simulink model "subsystem_118_bus_self_clearing_blocking"  (R2025b)
settings: Solver=ode45  StartTime=0.0  StopTime=Tstop  FixedStep=Ts  RelTol=1e-12  AbsTol=1e-12
values from neighbouring files (symbols this model uses):
  gfl3_enable_before = ones(numberOfGFLs,1)    [plotFun.m]
  gfl3_enable_blocked = gfl3_enable_before    [plotFun.m]
  gfl3_enable_clear_increment = gfl3_enable_before - gfl3_enable_blocked    [plotFun.m]
  gfl3_enable_zero = zeros(numberOfGFLs,1)    [plotFun.m]
  Imax = 15    [config_file.m]
  nominalInter =     [nominalInter.mat]
  nominalU =     [nominalU.mat]
  nominalY =     [nominalY.mat]
  P_input = 0    [main_sub_118_bus.m]    (also in plotFun.m = 0.03)
  sub = struct    [main_sub_118_bus.m]
  sys_j = sys_j(1:end-1)    [IBR_modelGenerator.m]
  sys_j_AA = sys_j    [modularMOR_main.m]
  sys_j_BT = sys_j    [modularMOR_main.m]
  Tclear_gfl = 0.11    [plotFun.m]
  Tstep_gfl = 0.1    [main_sub_118_bus.m]
  Tstep_gfm = 0.1    [main_sub_118_bus.m]
  Ttrip_gfl = 0.1    [plotFun.m]
  w = 2*pi*50    (= 314.159265359)    [config_file.m]    (also in mirrorMimoWeightedFrequencyData.m = w(:); modularMOR_main.m = w(:).'; plotTest.m = w(:).')
undefined symbols (not defined in the file or in its folder): con_sub, linSys1, linSys2, linSys3
libraries: simulink x10
(part 1 of 7)
settings Model: Creator=mj419  LastModifiedBy=hz1021
settings OptimizationCC: ReuseModelBlockBuffer=off
settings RTWCC: GPUComputeCapability=3.5

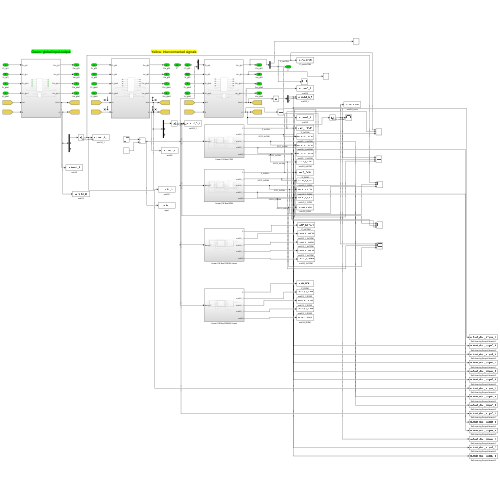
[thumbnail: Simulink's stored preview of the top-level diagram]
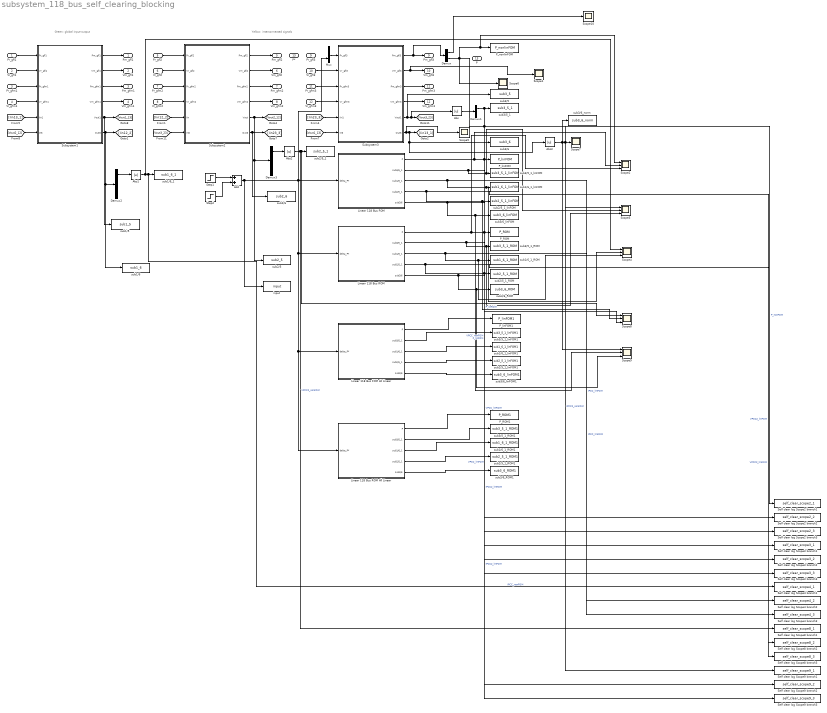
== system subsystem_118_bus_self_clearing_blocking ==
  note: Green: global input-output
  note: Yellow: interconnected signals
  Pr_gfl1 : Inport
  Vr_gfl1 : Inport  Port=2
  Pr_gfm1 : Inport  Port=3
  Vr_gfm1 : Inport  Port=4
  Pr_gfl2 : Inport  Port=5
  Vr_gfl2 : Inport  Port=6
  Pr_gfm2 : Inport  Port=7
  Vr_gfm2 : Inport  Port=8
  Pr_gfl3 : Inport  Port=9
  Vr_gfl3 : Inport  Port=10
  Pr_gfm3 : Inport  Port=11
  Vr_gfm3 : Inport  Port=12
  P* : Inport  Port=13
  Abs{,1..3} (4 alike) : Abs  SaturateOnIntegerOverflow=off
  Add : Sum
  Demux : Demux  Outputs=2
  Demux1 : Demux  Outputs=2
  Demux2 : Demux  Outputs=3
  Demux3 : Demux  Outputs=3
  Linear 118 Bus FOM : Subsystem
  Linear 118 Bus FOM All Linear : Subsystem
  Linear 118 Bus ROM : Subsystem
  Linear 118 Bus ROM All Linear : Subsystem
  Mux : Mux  Inputs=2
  P_ROM : ToWorkspace  VariableName=P_ROM  SaveFormat=Timeseries  SampleTime=-1
  P_ROM1 : ToWorkspace  VariableName=P_ROM1  SaveFormat=Timeseries  SampleTime=-1
  P_linFOM : ToWorkspace  VariableName=P_linFOM  SaveFormat=Timeseries  SampleTime=-1
  P_linFOM1 : ToWorkspace  VariableName=P_linFOM1  SaveFormat=Timeseries  SampleTime=-1
  P_nonlinFOM : ToWorkspace  VariableName=P_nonlinFOM  SaveFormat=Timeseries  SampleTime=-1
  Scope{1,5..7,10} (5 alike) : Scope
      Scope1 settings: ActiveDisplayYMinimum=1.0053183704569626  ActiveDisplayYMaximum=1.0729296783430808  DataLoggingVariableName=ScopeData4
      Scope10 settings: ActiveDisplayYMinimum=-0.0026208274368919567  ActiveDisplayYMaximum=0.0023961617330651047  DataLoggingVariableName=ScopeData13
      Scope5 settings: ActiveDisplayYMinimum=-0.10624375567453676  ActiveDisplayYMaximum=0.36712852641970622  DataLoggingVariableName=ScopeData8
      Scope6 settings: ActiveDisplayYMinimum=-0.0625349149097918  ActiveDisplayYMaximum=0.56250387943517355  DataLoggingVariableName=ScopeData9
      Scope7 settings: ActiveDisplayYMinimum=-0.0079180876925284485  ActiveDisplayYMaximum=0.35845618601099893  DataLoggingVariableName=ScopeData10
  Scope{2..4,8..9} (5 alike) : Scope  NumInputPorts=3
      Scope2 settings: ActiveDisplayYMinimum=-0.062546538096681009  ActiveDisplayYMaximum=0.56250517090103713  DataLoggingVariableName=ScopeData5
      Scope3 settings: ActiveDisplayYMinimum=0.81281465038704925  ActiveDisplayYMaximum=1.1717284729387976  DataLoggingVariableName=ScopeData6
      Scope4 settings: ActiveDisplayYMinimum=0.057385000514897075  ActiveDisplayYMaximum=0.10177777134395556  DataLoggingVariableName=ScopeData7
      Scope8 settings: ActiveDisplayYMinimum=1.0036213638969891  ActiveDisplayYMaximum=1.071548944692488  DataLoggingVariableName=ScopeData11
      Scope9 settings: ActiveDisplayYMinimum=-0.10716015389282768  ActiveDisplayYMaximum=0.37537611038432445  DataLoggingVariableName=ScopeData12
  Self clear log Scope2 branch1 : ToWorkspace  VariableName=self_clear_scope2_1  SaveFormat=Timeseries  SampleTime=-1
  Self clear log Scope2 branch2 : ToWorkspace  VariableName=self_clear_scope2_2  SaveFormat=Timeseries  SampleTime=-1
  Self clear log Scope2 branch3 : ToWorkspace  VariableName=self_clear_scope2_3  SaveFormat=Timeseries  SampleTime=-1
  Self clear log Scope3 branch1 : ToWorkspace  VariableName=self_clear_scope3_1  SaveFormat=Timeseries  SampleTime=-1
  Self clear log Scope3 branch2 : ToWorkspace  VariableName=self_clear_scope3_2  SaveFormat=Timeseries  SampleTime=-1
  Self clear log Scope3 branch3 : ToWorkspace  VariableName=self_clear_scope3_3  SaveFormat=Timeseries  SampleTime=-1
  Self clear log Scope4 branch1 : ToWorkspace  VariableName=self_clear_scope4_1  SaveFormat=Timeseries  SampleTime=-1
  Self clear log Scope4 branch2 : ToWorkspace  VariableName=self_clear_scope4_2  SaveFormat=Timeseries  SampleTime=-1
  Self clear log Scope4 branch3 : ToWorkspace  VariableName=self_clear_scope4_3  SaveFormat=Timeseries  SampleTime=-1
  Self clear log Scope8 branch1 : ToWorkspace  VariableName=self_clear_scope8_1  SaveFormat=Timeseries  SampleTime=-1
  Self clear log Scope8 branch2 : ToWorkspace  VariableName=self_clear_scope8_2  SaveFormat=Timeseries  SampleTime=-1
  Self clear log Scope8 branch3 : ToWorkspace  VariableName=self_clear_scope8_3  SaveFormat=Timeseries  SampleTime=-1
  Self clear log Scope9 branch1 : ToWorkspace  VariableName=self_clear_scope9_1  SaveFormat=Timeseries  SampleTime=-1
  Self clear log Scope9 branch2 : ToWorkspace  VariableName=self_clear_scope9_2  SaveFormat=Timeseries  SampleTime=-1
  Self clear log Scope9 branch3 : ToWorkspace  VariableName=self_clear_scope9_3  SaveFormat=Timeseries  SampleTime=-1
  Step1 : Step  Time=0.1  After=P_input  SampleTime=0
  Step2 : Step  Time=0.2  After=-0.02  SampleTime=0
  Subsystem1 : Subsystem
  Subsystem2 : Subsystem
  Subsystem3 : Subsystem
  input : ToWorkspace  VariableName=input  SaveFormat=Timeseries  SampleTime=-1
  sub1/5 : ToWorkspace  VariableName=sub1_5  SaveFormat=Timeseries  SampleTime=-1
  sub1/6 : ToWorkspace  VariableName=sub1_6  SaveFormat=Timeseries  SampleTime=-1
  sub1/6_1 : ToWorkspace  VariableName=sub1_6_1  SaveFormat=Timeseries  SampleTime=-1
  sub1/6_1_ROM : ToWorkspace  VariableName=sub1_6_1_ROM  SaveFormat=Timeseries  SampleTime=-1
  sub1/6_1_ROM1 : ToWorkspace  VariableName=sub1_6_1_ROM1  SaveFormat=Timeseries  SampleTime=-1
  sub1/6_1_linFOM : ToWorkspace  VariableName=sub1_6_1_linFOM  SaveFormat=Timeseries  SampleTime=-1
  sub1/6_1_linFOM1 : ToWorkspace  VariableName=sub1_6_1_linFOM1  SaveFormat=Timeseries  SampleTime=-1
  sub2/5 : ToWorkspace  VariableName=sub2_5  SaveFormat=Timeseries  SampleTime=-1
  sub2/5_1 : ToWorkspace  VariableName=sub2_5_1  SaveFormat=Timeseries  SampleTime=-1
  sub2/5_1_ROM : ToWorkspace  VariableName=sub2_5_1_ROM  SaveFormat=Timeseries  SampleTime=-1
  sub2/5_1_ROM1 : ToWorkspace  VariableName=sub2_5_1_ROM1  SaveFormat=Timeseries  SampleTime=-1
  sub2/5_1_linFOM : ToWorkspace  VariableName=sub2_5_1_linFOM  SaveFormat=Timeseries  SampleTime=-1
  sub2/5_1_linFOM1 : ToWorkspace  VariableName=sub2_5_1_linFOM1  SaveFormat=Timeseries  SampleTime=-1
  sub2/6 : ToWorkspace  VariableName=sub2_6  SaveFormat=Timeseries  SampleTime=-1
  sub3/5 : ToWorkspace  VariableName=sub3_5  SaveFormat=Timeseries  SampleTime=-1
  sub3/5_1 : ToWorkspace  VariableName=sub3_5_1  SaveFormat=Timeseries  SampleTime=-1
  sub3/5_1_ROM : ToWorkspace  VariableName=sub3_5_1_ROM  SaveFormat=Timeseries  SampleTime=-1
  sub3/5_1_ROM1 : ToWorkspace  VariableName=sub3_5_1_ROM1  SaveFormat=Timeseries  SampleTime=-1
  sub3/5_1_linFOM : ToWorkspace  VariableName=sub3_5_1_linFOM  SaveFormat=Timeseries  SampleTime=-1
  sub3/5_1_linFOM1 : ToWorkspace  VariableName=sub3_5_1_linFOM1  SaveFormat=Timeseries  SampleTime=-1
  sub3/6 : ToWorkspace  VariableName=sub3_6  SaveFormat=Timeseries  SampleTime=-1
  sub3/6_ROM : ToWorkspace  VariableName=sub3_6_ROM  SaveFormat=Timeseries  SampleTime=-1
  sub3/6_ROM1 : ToWorkspace  VariableName=sub3_6_ROM1  SaveFormat=Timeseries  SampleTime=-1
  sub3/6_linFOM : ToWorkspace  VariableName=sub3_6_linFOM  SaveFormat=Timeseries  SampleTime=-1
  sub3/6_linFOM1 : ToWorkspace  VariableName=sub3_6_linFOM1  SaveFormat=Timeseries  SampleTime=-1
  sub3/6_norm : ToWorkspace  VariableName=sub3_6_norm  SaveFormat=Timeseries  SampleTime=-1
  Pm_gfl1 : Outport
  Vm_gfl1 : Outport  Port=2
  Pm_gfm1 : Outport  Port=3
  Vm_gfm1 : Outport  Port=4
  Pm_gfl2 : Outport  Port=5
  Vm_gfl2 : Outport  Port=6
  Pm_gfm2 : Outport  Port=7
  Vm_gfm2 : Outport  Port=8
  Pm_gfl3 : Outport  Port=9
  Vm_gfl3 : Outport  Port=10
  Pm_gfm3 : Outport  Port=11
  Vm_gfm3 : Outport  Port=12
  P : Outport  Port=13
  wires:
  Pr_gfl1/1 -> Subsystem1/1(Pr_gfl1)
  Vr_gfl1/1 -> Subsystem1/2(Vr_gfl1)
  Pr_gfm1/1 -> Subsystem1/3(Pr_gfm1)
  Vr_gfm1/1 -> Subsystem1/4(Vr_gfm1)
  [Iin13_1] -> Subsystem1/5(Iin1)
  [Vout2_12] -> Subsystem1/6(In6)
  Subsystem1/1(Pm_gfl1) -> Pm_gfl1/1
  Subsystem1/2(Vm_gfl1) -> Vm_gfl1/1
  Subsystem1/3(Pm_gfm1) -> Pm_gfm1/1
  Subsystem1/4(Vm_gfm1) -> Vm_gfm1/1
  Subsystem1/6(Out6) -> sub1/6/1, Demux2/1, [Iin12_2]
  Pr_gfl2/1 -> Subsystem2/1(Pr_gfl2)
  Vr_gfl2/1 -> Subsystem2/2(Vr_gfl2)
  Pr_gfm2/1 -> Subsystem2/3(Pr_gfm2)
  Vr_gfm2/1 -> Subsystem2/4(Vr_gfm2)
  [Iin12_2] -> Subsystem2/5(Iin)
  [Vout3_23] -> Subsystem2/6(In6)
  Subsystem2/1(Pm_gfl2) -> Pm_gfl2/1
  Subsystem2/2(Vm_gfl2) -> Vm_gfl2/1
  Subsystem2/3(Pm_gfm2) -> Pm_gfm2/1
  Subsystem2/4(Vm_gfm2) -> Vm_gfm2/1
  Subsystem2/5(Vout) -> [Vout2_12], sub2/5/1, Demux3/1
  Subsystem2/6(Out6) -> sub2/6/1, [Iin23_3]
  [Iin23_3] -> Subsystem3/5(Iin1)
  [Vout1_13] -> Subsystem3/6(In6)
  Subsystem3/1(Pm_gfl3) -> Demux/1, Pm_gfl3/1
  Subsystem3/2(Vm_gfl3) -> Scope1/1, Vm_gfl3/1
  Subsystem3/3(Pm_gfm3) -> Pm_gfm3/1
  Subsystem3/4(Vm_gfm3) -> Vm_gfm3/1
  Subsystem3/5(Vout1) -> sub3/5/1, Abs/1, [Vout3_23]
  Subsystem3/6(Out6) -> Scope5/1, Abs3/1, sub3/6/1, [Iin13_1]
  Pr_gfm3/1 -> Subsystem3/3(Pr_gfm3)
  Vr_gfm3/1 -> Subsystem3/4(Vr_gfm3)
  Vr_gfl3/1 -> Subsystem3/2(Vr_gfl3)
  Mux/1 -> Subsystem3/1(Pr_gfl3)
  Abs/1 -> Demux1/1
  Demux1/1 -> Self clear log Scope3 branch1/1, Scope3/1, sub3/5_1/1  "VPCC_nonFOM"
  Linear 118 Bus ROM/1(P) -> Self clear log Scope2 branch3/1, P_ROM/1, Scope2/3  "P_linROM"
  Linear 118 Bus FOM/1(P) -> Self clear log Scope2 branch2/1, P_linFOM/1, Scope2/2  "P_linFOM"
  Demux/2 -> Self clear log Scope2 branch1/1, Scope6/1, Scope2/1, P_nonlinFOM/1  "P_nonFOM"
  Linear 118 Bus ROM/2(sub3/5_1) -> Scope3/3, sub3/5_1_ROM/1, Self clear log Scope3 branch3/1  "VPCC_linROM"
  Subsystem1/5(Vout1) -> [Vout1_13], sub1/5/1
  Linear 118 Bus ROM/3(sub1/6_1) -> sub1/6_1_ROM/1, Scope4/3, Self clear log Scope4 branch3/1  "IPCC_linROM"
  Linear 118 Bus ROM/4(sub2/5_1) -> sub2/5_1_ROM/1, Scope8/3, Self clear log Scope8 branch3/1  "VPCC2_linROM"
  Linear 118 Bus FOM/2(sub3/5_1) -> Scope3/2, sub3/5_1_linFOM/1, Self clear log Scope3 branch2/1  "VPCC_linFOM"
  Linear 118 Bus FOM/3(sub1/6_1) -> Scope4/2, sub1/6_1_linFOM/1, Self clear log Scope4 branch2/1  "IPCC_linFOM"
  Linear 118 Bus FOM/4(sub2/5_1) -> sub2/5_1_linFOM/1, Scope8/2, Self clear log Scope8 branch2/1  "VPCC2_linFOM"
  Demux2/1 -> Abs1/1
  Abs1/1 -> Self clear log Scope4 branch1/1, sub1/6_1/1, Scope4/1  "IPCC_nonFOM"
  Demux3/1 -> Abs2/1
  Abs2/1 -> Scope8/1, sub2/5_1/1, Self clear log Scope8 branch1/1  "VPCC2_nonFOM"
  Abs3/1 -> Self clear log Scope9 branch1/1, Scope7/1, sub3/6_norm/1, Scope9/1  "IPCC2_nonFOM"
  Linear 118 Bus ROM/5(sub3/6) -> sub3/6_ROM/1, Scope9/3, Self clear log Scope9 branch3/1  "IPCC2_linROM"
  Linear 118 Bus FOM/5(sub3/6) -> sub3/6_linFOM/1, Scope9/2, Self clear log Scope9 branch2/1  "IPCC2_linFOM"
  Step2/1 -> Add/2
  Add/1 -> input/1, Mux/2, Linear 118 Bus ROM All Linear/1(delta_P*), Linear 118 Bus FOM All Linear/1(delta_P*), Linear 118 Bus ROM/1(delta_P*), Linear 118 Bus FOM/1(delta_P*)
  Step1/1 -> Add/1
  Linear 118 Bus ROM All Linear/1(P) -> P_ROM1/1
  Linear 118 Bus ROM All Linear/2(sub3/5_1) -> sub3/5_1_ROM1/1
  Linear 118 Bus ROM All Linear/3(sub1/6_1) -> sub1/6_1_ROM1/1
  Linear 118 Bus ROM All Linear/4(sub2/5_1) -> sub2/5_1_ROM1/1
  Linear 118 Bus ROM All Linear/5(sub3/6) -> sub3/6_ROM1/1
  Linear 118 Bus FOM All Linear/1(P) -> P_linFOM1/1
  Linear 118 Bus FOM All Linear/2(sub3/5_1) -> sub3/5_1_linFOM1/1
  Linear 118 Bus FOM All Linear/3(sub1/6_1) -> sub1/6_1_linFOM1/1
  Linear 118 Bus FOM All Linear/4(sub2/5_1) -> sub2/5_1_linFOM1/1
  Linear 118 Bus FOM All Linear/5(sub3/6) -> sub3/6_linFOM1/1
  Demux/1 -> Scope10/1

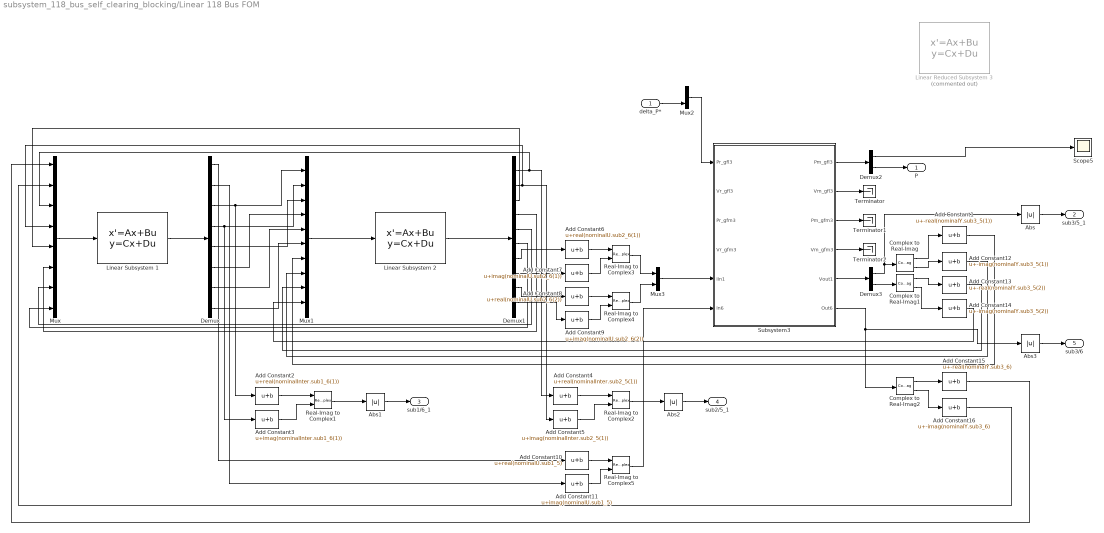
== system subsystem_118_bus_self_clearing_blocking/Linear 118 Bus FOM ==
  delta_P* : Inport
  Abs{,1..3} (4 alike) : Abs  SaturateOnIntegerOverflow=off
  Add Constant1 : Bias  Bias=-real(nominalY.sub3_5(1))  SaturateOnIntegerOverflow=off
  Add Constant10 : Bias  Bias=real(nominalU.sub1_5)  SaturateOnIntegerOverflow=off
  Add Constant11 : Bias  Bias=imag(nominalU.sub1_5)  SaturateOnIntegerOverflow=off
  Add Constant12 : Bias  Bias=-imag(nominalY.sub3_5(1))  SaturateOnIntegerOverflow=off
  Add Constant13 : Bias  Bias=-real(nominalY.sub3_5(2))  SaturateOnIntegerOverflow=off
  Add Constant14 : Bias  Bias=-imag(nominalY.sub3_5(2))  SaturateOnIntegerOverflow=off
  Add Constant15 : Bias  Bias=-real(nominalY.sub3_6)  SaturateOnIntegerOverflow=off
  Add Constant16 : Bias  Bias=-imag(nominalY.sub3_6)  SaturateOnIntegerOverflow=off
  Add Constant2 : Bias  Bias=real(nominalInter.sub1_6(1))  SaturateOnIntegerOverflow=off
  Add Constant3 : Bias  Bias=imag(nominalInter.sub1_6(1))  SaturateOnIntegerOverflow=off
  Add Constant4 : Bias  Bias=real(nominalInter.sub2_5(1))  SaturateOnIntegerOverflow=off
  Add Constant5 : Bias  Bias=imag(nominalInter.sub2_5(1))  SaturateOnIntegerOverflow=off
  Add Constant6 : Bias  Bias=real(nominalU.sub2_6(1))  SaturateOnIntegerOverflow=off
  Add Constant7 : Bias  Bias=imag(nominalU.sub2_6(1))  SaturateOnIntegerOverflow=off
  Add Constant8 : Bias  Bias=real(nominalU.sub2_6(2))  SaturateOnIntegerOverflow=off
  Add Constant9 : Bias  Bias=imag(nominalU.sub2_6(2))  SaturateOnIntegerOverflow=off
  Complex to Real-Imag : ComplexToRealImag
  Complex to Real-Imag1 : ComplexToRealImag
  Complex to Real-Imag2 : ComplexToRealImag
  Demux : Demux  Outputs=8
  Demux1 : Demux  Outputs=10
  Demux2 : Demux  Outputs=2
  Demux3 : Demux  Outputs=2
  Linear Reduced Subsystem 3 : StateSpace  Commented=on  A=sys_j(3).rss.A  B=sys_j(3).rss.B  C=sys_j(3).rss.C  D=sys_j(3).rss.D  InitialCondition=0
  Linear Subsystem 1 : StateSpace  A=linSys1.A  B=linSys1.B  C=linSys1.C  D=linSys1.D  InitialCondition=0
  Linear Subsystem 2 : StateSpace  A=linSys2.A  B=linSys2.B  C=linSys2.C  D=linSys2.D  InitialCondition=0
  Mux : Mux  Inputs=8
  Mux1 : Mux  Inputs=10
  Mux2 : Mux  Inputs=2
  Mux3 : Mux  Inputs=2
  Real-Imag to Complex{1..5} (5 alike) : RealImagToComplex
  Scope5 : Scope
      settings: ActiveDisplayYMinimum=-0.0030129134761664742  ActiveDisplayYMaximum=0.0027387712384938576  DataLoggingVariableName=ScopeData14
  Subsystem3 : Subsystem
  Terminator : Terminator
  Terminator1 : Terminator
  Terminator2 : Terminator
  P : Outport
  sub3/5_1 : Outport  Port=2
  sub1/6_1 : Outport  Port=3
  sub2/5_1 : Outport  Port=4
  sub3/6 : Outport  Port=5
  wires:
  Demux/3 -> Add Constant2/1, Mux1/1
  Demux1/6 -> Mux/8
  Demux/8 -> Mux1/6
  Demux1/2 -> Mux/4, Add Constant5/1
  Demux/4 -> Add Constant3/1, Mux1/2
  Demux1/1 -> Add Constant4/1, Mux/3
  Demux1/3 -> Mux/5
  Demux1/5 -> Mux/7
  Demux/6 -> Mux1/4
  Demux/7 -> Mux1/5
  Demux1/4 -> Mux/6
  Demux/5 -> Mux1/3
  Mux1/1 -> Linear Subsystem 2/1
  Mux/1 -> Linear Subsystem 1/1
  Linear Subsystem 1/1 -> Demux/1
  Linear Subsystem 2/1 -> Demux1/1
  Abs/1 -> sub3/5_1/1
  Add Constant3/1 -> Real-Imag to Complex1/2
  Add Constant2/1 -> Real-Imag to Complex1/1
  Real-Imag to Complex1/1 -> Abs1/1
  Abs1/1 -> sub1/6_1/1
  Add Constant5/1 -> Real-Imag to Complex2/2
  Add Constant4/1 -> Real-Imag to Complex2/1
  Real-Imag to Complex2/1 -> Abs2/1
  Abs2/1 -> sub2/5_1/1
  delta_P*/1 -> Mux2/2
  Mux2/1 -> Subsystem3/1(Pr_gfl3)
  Demux1/7 -> Add Constant6/1
  Demux1/8 -> Add Constant7/1
  Demux1/9 -> Add Constant8/1
  Demux1/10 -> Add Constant9/1
  Add Constant6/1 -> Real-Imag to Complex3/1
  Add Constant7/1 -> Real-Imag to Complex3/2
  Add Constant8/1 -> Real-Imag to Complex4/1
  Add Constant9/1 -> Real-Imag to Complex4/2
  Real-Imag to Complex3/1 -> Mux3/1
  Real-Imag to Complex4/1 -> Mux3/2
  Mux3/1 -> Subsystem3/5(Iin1)
  Add Constant11/1 -> Real-Imag to Complex5/2
  Real-Imag to Complex5/1 -> Subsystem3/6(In6)
  Demux/2 -> Add Constant11/1
  Add Constant10/1 -> Real-Imag to Complex5/1
  Demux/1 -> Add Constant10/1
  Subsystem3/1(Pm_gfl3) -> Demux2/1
  Demux2/2 -> P/1
  Subsystem3/5(Vout1) -> Demux3/1
  Demux3/1 -> Complex to Real-Imag/1, Abs/1
  Demux3/2 -> Complex to Real-Imag1/1
  Complex to Real-Imag/1 -> Add Constant1/1
  Complex to Real-Imag/2 -> Add Constant12/1
  Complex to Real-Imag1/1 -> Add Constant13/1
  Complex to Real-Imag1/2 -> Add Constant14/1
  Add Constant1/1 -> Mux1/7
  Add Constant12/1 -> Mux1/8
  Add Constant13/1 -> Mux1/9
  Add Constant14/1 -> Mux1/10
  Complex to Real-Imag2/1 -> Add Constant15/1
  Complex to Real-Imag2/2 -> Add Constant16/1
  Add Constant15/1 -> Mux/1
  Add Constant16/1 -> Mux/2
  Subsystem3/2(Vm_gfl3) -> Terminator/1
  Subsystem3/3(Pm_gfm3) -> Terminator1/1
  Subsystem3/4(Vm_gfm3) -> Terminator2/1
  Subsystem3/6(Out6) -> Abs3/1, Complex to Real-Imag2/1
  Abs3/1 -> sub3/6/1
  Demux2/1 -> Scope5/1

== system subsystem_118_bus_self_clearing_blocking/Linear 118 Bus FOM All Linear ==
  delta_P* : Inport
  Abs{,1..3} (4 alike) : Abs  SaturateOnIntegerOverflow=off
  Add Constant1 : Bias  Bias=real(nominalY.sub3_5(1))  SaturateOnIntegerOverflow=off
  Add Constant12 : Bias  Bias=imag(nominalY.sub3_5(1))  SaturateOnIntegerOverflow=off
  Add Constant15 : Bias  Bias=real(nominalY.sub3_6)  SaturateOnIntegerOverflow=off
  Add Constant16 : Bias  Bias=imag(nominalY.sub3_6)  SaturateOnIntegerOverflow=off
  Add Constant2 : Bias  Bias=real(nominalInter.sub1_6(1))  SaturateOnIntegerOverflow=off
  Add Constant3 : Bias  Bias=imag(nominalInter.sub1_6(1))  SaturateOnIntegerOverflow=off
  Add Constant4 : Bias  Bias=real(nominalInter.sub2_5(1))  SaturateOnIntegerOverflow=off
  Add Constant5 : Bias  Bias=imag(nominalInter.sub2_5(1))  SaturateOnIntegerOverflow=off
  Add Constant6 : Bias  Bias=nominalY.P  SaturateOnIntegerOverflow=off
  Demux : Demux  Outputs=8
  Demux1 : Demux  Outputs=10
  Demux2 : Demux  Outputs=7
  Linear Subsystem 1 : StateSpace  A=linSys1.A  B=linSys1.B  C=linSys1.C  D=linSys1.D  InitialCondition=0
  Linear Subsystem 2 : StateSpace  A=linSys2.A  B=linSys2.B  C=linSys2.C  D=linSys2.D  InitialCondition=0
  Linear Subsystem 3 : StateSpace  A=linSys3.A  B=linSys3.B  C=linSys3.C  D=linSys3.D  InitialCondition=0
  Mux : Mux  Inputs=8
  Mux1 : Mux  Inputs=10
  Mux2 : Mux  Inputs=7
  Real-Imag to Complex{1..4} (4 alike) : RealImagToComplex
  P : Outport
  sub3/5_1 : Outport  Port=2
  sub1/6_1 : Outport  Port=3
  sub2/5_1 : Outport  Port=4
  sub3/6 : Outport  Port=5
  wires:
  Demux/3 -> Add Constant2/1, Mux1/1
  Demux1/6 -> Mux/8
  Demux/1 -> Mux2/5
  Demux/8 -> Mux1/6
  Demux1/2 -> Add Constant5/1, Mux/4
  Demux/4 -> Add Constant3/1, Mux1/2
  Demux1/1 -> Add Constant4/1, Mux/3
  Demux1/7 -> Mux2/1
  Demux1/3 -> Mux/5
  Demux1/5 -> Mux/7
  delta_P*/1 -> Mux2/7
  Demux2/3 -> Add Constant12/1, Mux1/8
  Demux/6 -> Mux1/4
  Demux/7 -> Mux1/5
  Demux2/4 -> Mux1/9
  Demux2/2 -> Mux1/7, Add Constant1/1
  Demux1/4 -> Mux/6
  Demux1/9 -> Mux2/3
  Demux/5 -> Mux1/3
  Demux2/7 -> Add Constant16/1, Mux/2
  Mux1/1 -> Linear Subsystem 2/1
  Demux2/6 -> Add Constant15/1, Mux/1
  Mux/1 -> Linear Subsystem 1/1
  Demux1/8 -> Mux2/2
  Demux/2 -> Mux2/6
  Demux2/5 -> Mux1/10
  Demux1/10 -> Mux2/4
  Linear Subsystem 1/1 -> Demux/1
  Mux2/1 -> Linear Subsystem 3/1
  Linear Subsystem 2/1 -> Demux1/1
  Linear Subsystem 3/1 -> Demux2/1
  Real-Imag to Complex2/1 -> Abs/1
  Abs/1 -> sub3/5_1/1
  Add Constant15/1 -> Real-Imag to Complex1/1
  Add Constant16/1 -> Real-Imag to Complex1/2
  Real-Imag to Complex1/1 -> Abs1/1
  Abs1/1 -> sub3/6/1
  Add Constant1/1 -> Real-Imag to Complex2/1
  Add Constant12/1 -> Real-Imag to Complex2/2
  Add Constant3/1 -> Real-Imag to Complex3/2
  Abs2/1 -> sub1/6_1/1
  Real-Imag to Complex3/1 -> Abs2/1
  Add Constant2/1 -> Real-Imag to Complex3/1
  Add Constant5/1 -> Real-Imag to Complex4/2
  Abs3/1 -> sub2/5_1/1
  Add Constant4/1 -> Real-Imag to Complex4/1
  Real-Imag to Complex4/1 -> Abs3/1
  Demux2/1 -> Add Constant6/1
  Add Constant6/1 -> P/1

== system subsystem_118_bus_self_clearing_blocking/Linear 118 Bus ROM ==
  delta_P* : Inport
  Abs{,1..3} (4 alike) : Abs  SaturateOnIntegerOverflow=off
  Add Constant1 : Bias  Bias=-real(nominalY.sub3_5(1))  SaturateOnIntegerOverflow=off
  Add Constant10 : Bias  Bias=real(nominalU.sub1_5)  SaturateOnIntegerOverflow=off
  Add Constant11 : Bias  Bias=imag(nominalU.sub1_5)  SaturateOnIntegerOverflow=off
  Add Constant12 : Bias  Bias=-imag(nominalY.sub3_5(1))  SaturateOnIntegerOverflow=off
  Add Constant13 : Bias  Bias=-real(nominalY.sub3_5(2))  SaturateOnIntegerOverflow=off
  Add Constant14 : Bias  Bias=-imag(nominalY.sub3_5(2))  SaturateOnIntegerOverflow=off
  Add Constant15 : Bias  Bias=-real(nominalY.sub3_6)  SaturateOnIntegerOverflow=off
  Add Constant16 : Bias  Bias=-imag(nominalY.sub3_6)  SaturateOnIntegerOverflow=off
  Add Constant2 : Bias  Bias=real(nominalInter.sub1_6(1))  SaturateOnIntegerOverflow=off
  Add Constant3 : Bias  Bias=imag(nominalInter.sub1_6(1))  SaturateOnIntegerOverflow=off
  Add Constant4 : Bias  Bias=real(nominalInter.sub2_5(1))  SaturateOnIntegerOverflow=off
  Add Constant5 : Bias  Bias=imag(nominalInter.sub2_5(1))  SaturateOnIntegerOverflow=off
  Add Constant6 : Bias  Bias=real(nominalU.sub2_6(1))  SaturateOnIntegerOverflow=off
  Add Constant7 : Bias  Bias=imag(nominalU.sub2_6(1))  SaturateOnIntegerOverflow=off
  Add Constant8 : Bias  Bias=real(nominalU.sub2_6(2))  SaturateOnIntegerOverflow=off
  Add Constant9 : Bias  Bias=imag(nominalU.sub2_6(2))  SaturateOnIntegerOverflow=off
  Complex to Real-Imag : ComplexToRealImag
  Complex to Real-Imag1 : ComplexToRealImag
  Complex to Real-Imag2 : ComplexToRealImag
  Demux : Demux  Outputs=8
  Demux1 : Demux  Outputs=10
  Demux2 : Demux  Outputs=2
  Demux3 : Demux  Outputs=2
  Linear Reduced Subsystem 1 : StateSpace  A=sys_j_BT(1).rss.A  B=sys_j_BT(1).rss.B  C=sys_j_BT(1).rss.C  D=sys_j_BT(1).rss.D  InitialCondition=0
  Linear Reduced Subsystem 2 : StateSpace  A=sys_j_AA(2).rss.A  B=sys_j_AA(2).rss.B  C=sys_j_AA(2).rss.C  D=sys_j_AA(2).rss.D  InitialCondition=0
  Linear Reduced Subsystem 3 : StateSpace  Commented=on  A=sys_j(3).rss.A  B=sys_j(3).rss.B  C=sys_j(3).rss.C  D=sys_j(3).rss.D  InitialCondition=0
  Mux : Mux  Inputs=8
  Mux1 : Mux  Inputs=10
  Mux2 : Mux  Inputs=2
  Mux3 : Mux  Inputs=2
  Real-Imag to Complex{1..5} (5 alike) : RealImagToComplex
  Scope5 : Scope
      settings: ActiveDisplayYMinimum=-0.0029327482221316362  ActiveDisplayYMaximum=0.0026650174766488623  DataLoggingVariableName=ScopeData15
  Subsystem3 : Subsystem
  Terminator : Terminator
  Terminator1 : Terminator
  Terminator2 : Terminator
  P : Outport
  sub3/5_1 : Outport  Port=2
  sub1/6_1 : Outport  Port=3
  sub2/5_1 : Outport  Port=4
  sub3/6 : Outport  Port=5
  wires:
  Demux/3 -> Add Constant2/1, Mux1/1
  Demux1/6 -> Mux/8
  Demux/8 -> Mux1/6
  Demux1/2 -> Mux/4, Add Constant5/1
  Demux/4 -> Add Constant3/1, Mux1/2
  Demux1/1 -> Add Constant4/1, Mux/3
  Demux1/3 -> Mux/5
  Demux1/5 -> Mux/7
  Demux/6 -> Mux1/4
  Demux/7 -> Mux1/5
  Demux1/4 -> Mux/6
  Demux/5 -> Mux1/3
  Mux1/1 -> Linear Reduced Subsystem 2/1
  Mux/1 -> Linear Reduced Subsystem 1/1
  Linear Reduced Subsystem 1/1 -> Demux/1
  Linear Reduced Subsystem 2/1 -> Demux1/1
  Abs/1 -> sub3/5_1/1
  Add Constant3/1 -> Real-Imag to Complex1/2
  Add Constant2/1 -> Real-Imag to Complex1/1
  Real-Imag to Complex1/1 -> Abs1/1
  Abs1/1 -> sub1/6_1/1
  Add Constant5/1 -> Real-Imag to Complex2/2
  Add Constant4/1 -> Real-Imag to Complex2/1
  Real-Imag to Complex2/1 -> Abs2/1
  Abs2/1 -> sub2/5_1/1
  delta_P*/1 -> Mux2/2
  Mux2/1 -> Subsystem3/1(Pr_gfl3)
  Demux1/7 -> Add Constant6/1
  Demux1/8 -> Add Constant7/1
  Demux1/9 -> Add Constant8/1
  Demux1/10 -> Add Constant9/1
  Add Constant6/1 -> Real-Imag to Complex3/1
  Add Constant7/1 -> Real-Imag to Complex3/2
  Add Constant8/1 -> Real-Imag to Complex4/1
  Add Constant9/1 -> Real-Imag to Complex4/2
  Real-Imag to Complex3/1 -> Mux3/1
  Real-Imag to Complex4/1 -> Mux3/2
  Mux3/1 -> Subsystem3/5(Iin1)
  Add Constant11/1 -> Real-Imag to Complex5/2
  Real-Imag to Complex5/1 -> Subsystem3/6(In6)
  Demux/2 -> Add Constant11/1
  Add Constant10/1 -> Real-Imag to Complex5/1
  Demux/1 -> Add Constant10/1
  Subsystem3/1(Pm_gfl3) -> Demux2/1
  Demux2/2 -> P/1
  Subsystem3/5(Vout1) -> Demux3/1
  Demux3/1 -> Complex to Real-Imag/1, Abs/1
  Demux3/2 -> Complex to Real-Imag1/1
  Complex to Real-Imag/1 -> Add Constant1/1
  Complex to Real-Imag/2 -> Add Constant12/1
  Complex to Real-Imag1/1 -> Add Constant13/1
  Complex to Real-Imag1/2 -> Add Constant14/1
  Add Constant1/1 -> Mux1/7
  Add Constant12/1 -> Mux1/8
  Add Constant13/1 -> Mux1/9
  Add Constant14/1 -> Mux1/10
  Subsystem3/6(Out6) -> Abs3/1, Complex to Real-Imag2/1
  Complex to Real-Imag2/1 -> Add Constant15/1
  Complex to Real-Imag2/2 -> Add Constant16/1
  Add Constant15/1 -> Mux/1
  Add Constant16/1 -> Mux/2
  Subsystem3/2(Vm_gfl3) -> Terminator/1
  Subsystem3/3(Pm_gfm3) -> Terminator1/1
  Subsystem3/4(Vm_gfm3) -> Terminator2/1
  Abs3/1 -> sub3/6/1
  Demux2/1 -> Scope5/1

== system subsystem_118_bus_self_clearing_blocking/Linear 118 Bus ROM All Linear ==
  delta_P* : Inport
  Abs{,1..3} (4 alike) : Abs  SaturateOnIntegerOverflow=off
  Add Constant1 : Bias  Bias=real(nominalY.sub3_5(1))  SaturateOnIntegerOverflow=off
  Add Constant12 : Bias  Bias=imag(nominalY.sub3_5(1))  SaturateOnIntegerOverflow=off
  Add Constant15 : Bias  Bias=real(nominalY.sub3_6)  SaturateOnIntegerOverflow=off
  Add Constant16 : Bias  Bias=imag(nominalY.sub3_6)  SaturateOnIntegerOverflow=off
  Add Constant2 : Bias  Bias=real(nominalInter.sub1_6(1))  SaturateOnIntegerOverflow=off
  Add Constant3 : Bias  Bias=imag(nominalInter.sub1_6(1))  SaturateOnIntegerOverflow=off
  Add Constant4 : Bias  Bias=real(nominalInter.sub2_5(1))  SaturateOnIntegerOverflow=off
  Add Constant5 : Bias  Bias=imag(nominalInter.sub2_5(1))  SaturateOnIntegerOverflow=off
  Add Constant6 : Bias  Bias=nominalY.P  SaturateOnIntegerOverflow=off
  Demux : Demux  Outputs=8
  Demux1 : Demux  Outputs=10
  Demux2 : Demux  Outputs=7
  Linear Reduced Subsystem 1 : StateSpace  A=sys_j_BT(1).rss.A  B=sys_j_BT(1).rss.B  C=sys_j_BT(1).rss.C  D=sys_j_BT(1).rss.D  InitialCondition=0
  Linear Reduced Subsystem 2 : StateSpace  A=sys_j_AA(2).rss.A  B=sys_j_AA(2).rss.B  C=sys_j_AA(2).rss.C  D=sys_j_AA(2).rss.D  InitialCondition=0
  Linear Reduced Subsystem 3 : StateSpace  A=linSys3.A  B=linSys3.B  C=linSys3.C  D=linSys3.D  InitialCondition=0
  Mux : Mux  Inputs=8
  Mux1 : Mux  Inputs=10
  Mux2 : Mux  Inputs=7
  Real-Imag to Complex{1..4} (4 alike) : RealImagToComplex
  P : Outport
  sub3/5_1 : Outport  Port=2
  sub1/6_1 : Outport  Port=3
  sub2/5_1 : Outport  Port=4
  sub3/6 : Outport  Port=5
  wires:
  Demux/3 -> Add Constant2/1, Mux1/1
  Demux1/6 -> Mux/8
  Demux/1 -> Mux2/5
  Demux/8 -> Mux1/6
  Demux1/2 -> Add Constant5/1, Mux/4
  Demux/4 -> Add Constant3/1, Mux1/2
  Demux1/1 -> Add Constant4/1, Mux/3
  Demux1/7 -> Mux2/1
  Demux1/3 -> Mux/5
  Demux1/5 -> Mux/7
  delta_P*/1 -> Mux2/7
  Demux2/3 -> Add Constant12/1, Mux1/8
  Demux/6 -> Mux1/4
  Demux/7 -> Mux1/5
  Demux2/4 -> Mux1/9
  Demux2/2 -> Mux1/7, Add Constant1/1
  Demux1/4 -> Mux/6
  Demux1/9 -> Mux2/3
  Demux/5 -> Mux1/3
  Demux2/7 -> Add Constant16/1, Mux/2
  Mux1/1 -> Linear Reduced Subsystem 2/1
  Demux2/6 -> Add Constant15/1, Mux/1
  Mux/1 -> Linear Reduced Subsystem 1/1
  Demux1/8 -> Mux2/2
  Demux/2 -> Mux2/6
  Demux2/5 -> Mux1/10
  Demux1/10 -> Mux2/4
  Linear Reduced Subsystem 1/1 -> Demux/1
  Mux2/1 -> Linear Reduced Subsystem 3/1
  Linear Reduced Subsystem 2/1 -> Demux1/1
  Linear Reduced Subsystem 3/1 -> Demux2/1
  Real-Imag to Complex2/1 -> Abs/1
  Abs/1 -> sub3/5_1/1
  Add Constant15/1 -> Real-Imag to Complex1/1
  Add Constant16/1 -> Real-Imag to Complex1/2
  Real-Imag to Complex1/1 -> Abs1/1
  Abs1/1 -> sub3/6/1
  Add Constant1/1 -> Real-Imag to Complex2/1
  Add Constant12/1 -> Real-Imag to Complex2/2
  Add Constant3/1 -> Real-Imag to Complex3/2
  Abs2/1 -> sub1/6_1/1
  Real-Imag to Complex3/1 -> Abs2/1
  Add Constant2/1 -> Real-Imag to Complex3/1
  Add Constant5/1 -> Real-Imag to Complex4/2
  Abs3/1 -> sub2/5_1/1
  Add Constant4/1 -> Real-Imag to Complex4/1
  Real-Imag to Complex4/1 -> Abs3/1
  Demux2/1 -> Add Constant6/1
  Add Constant6/1 -> P/1

== system subsystem_118_bus_self_clearing_blocking/Subsystem1 ==
  Pr_gfl1 : Inport
  Vr_gfl1 : Inport  Port=2
  Pr_gfm1 : Inport  Port=3
  Vr_gfm1 : Inport  Port=4
  Iin1 : Inport  Port=5
  In6 : Inport  Port=6
  area1 : Subsystem  mask{Subsystem=sub(1)}
      mask prompts: Subsystem "Struct"
      mask Display: disp(get_param(gcb,'Subsystem'));
  con12 : Subsystem  mask{con_subsystem=con_sub(1)}
      mask prompts: con_subsystem "Struct"
      mask Display: disp(get_param(gcb,'con_subsystem'));
  Pm_gfl1 : Outport
  Vm_gfl1 : Outport  Port=2
  Pm_gfm1 : Outport  Port=3
  Vm_gfm1 : Outport  Port=4
  Vout1 : Outport  Port=5
  Out6 : Outport  Port=6
  wires:
  area1/3(Pm_gfm) -> Pm_gfm1/1
  area1/5(Vout) -> [Vout1_12]
  Vr_gfl1/1 -> area1/2(Vr_gfl)
  con12/2(Out2) -> Out6/1
  con12/1(Out1) -> [Iin12_1]
  area1/2(Vm_gfl) -> Vm_gfl1/1
  Pr_gfl1/1 -> area1/1(Pr_gfl)
  area1/1(Pm_gfl) -> Pm_gfl1/1
  [Vout1_12] -> con12/1(In1)
  [Iin12_1] -> area1/5(Iin)
  Vr_gfm1/1 -> area1/4(Vr_gfm)
  Pr_gfm1/1 -> area1/3(Pr_gfm)
  area1/4(Vm_gfm) -> Vm_gfm1/1
  In6/1 -> con12/2(In2)
  area1/6(Vout1) -> Vout1/1
  Iin1/1 -> area1/6(Iin1)

== system subsystem_118_bus_self_clearing_blocking/Subsystem2 ==
  Pr_gfl2 : Inport
  Vr_gfl2 : Inport  Port=2
  Pr_gfm2 : Inport  Port=3
  Vr_gfm2 : Inport  Port=4
  Iin : Inport  Port=5
  In6 : Inport  Port=6
  area2 : Subsystem  mask{Subsystem=sub(2)}
      mask prompts: Subsystem "Struct"
      mask Display: disp(get_param(gcb,'Subsystem'));
  con23 : Subsystem  mask{con_subsystem=con_sub(3)}
      mask prompts: con_subsystem "Struct"
      mask Display: disp(get_param(gcb,'con_subsystem'));
  Pm_gfl2 : Outport
  Vm_gfl2 : Outport  Port=2
  Pm_gfm2 : Outport  Port=3
  Vm_gfm2 : Outport  Port=4
  Vout : Outport  Port=5
  Out6 : Outport  Port=6
  wires:
  [Iin23_2] -> area2/6(Iin1)
  area2/6(Vout1) -> [Vout2_23]
  Vr_gfm2/1 -> area2/4(Vr_gfm)
  Pr_gfl2/1 -> area2/1(Pr_gfl)
  con23/1(Out1) -> [Iin23_2]
  area2/4(Vm_gfm) -> Vm_gfm2/1
  Pr_gfm2/1 -> area2/3(Pr_gfm)
  [Vout2_23] -> con23/1(In1)
  area2/3(Pm_gfm) -> Pm_gfm2/1
  Vr_gfl2/1 -> area2/2(Vr_gfl)
  area2/2(Vm_gfl) -> Vm_gfl2/1
  area2/1(Pm_gfl) -> Pm_gfl2/1
  area2/5(Vout) -> Vout/1
  Iin/1 -> area2/5(Iin)
  con23/2(Out2) -> Out6/1
  In6/1 -> con23/2(In2)

== system subsystem_118_bus_self_clearing_blocking/Subsystem3 ==
  Pr_gfl3 : Inport
  Vr_gfl3 : Inport  Port=2
  Pr_gfm3 : Inport  Port=3
  Vr_gfm3 : Inport  Port=4
  Iin1 : Inport  Port=5
  In6 : Inport  Port=6
  area3 : Subsystem  mask{Subsystem=sub(3)}
      mask prompts: Subsystem "Struct"
      mask Display: disp(get_param(gcb,'Subsystem'));
  con13 : Subsystem  mask{con_subsystem=con_sub(2)}
      mask prompts: con_subsystem "Struct"
      mask Display: disp(get_param(gcb,'con_subsystem'));
  Pm_gfl3 : Outport
  Vm_gfl3 : Outport  Port=2
  Pm_gfm3 : Outport  Port=3
  Vm_gfm3 : Outport  Port=4
  Vout1 : Outport  Port=5
  Out6 : Outport  Port=6
  wires:
  con13/2(Out2) -> [Iin13_3]
  area3/5(Vout) -> [Vout3_13]
  [Vout3_13] -> con13/2(In2)
  Vr_gfm3/1 -> area3/4(Vr_gfm)
  [Iin13_3] -> area3/5(Iin)
  Vr_gfl3/1 -> area3/2(Vr_gfl)
  Pr_gfl3/1 -> area3/1(Pr_gfl)
  area3/6(Vout1) -> Vout1/1
  Pr_gfm3/1 -> area3/3(Pr_gfm)
  area3/1(Pm_gfl) -> Pm_gfl3/1
  area3/2(Vm_gfl) -> Vm_gfl3/1
  area3/4(Vm_gfm) -> Vm_gfm3/1
  area3/3(Pm_gfm) -> Pm_gfm3/1
  con13/1(Out1) -> Out6/1
  Iin1/1 -> area3/6(Iin1)
  In6/1 -> con13/1(In1)

== system subsystem_118_bus_self_clearing_blocking/Linear 118 Bus FOM/Subsystem3 ==
  Pr_gfl3 : Inport
  Vr_gfl3 : Inport  Port=2
  Pr_gfm3 : Inport  Port=3
  Vr_gfm3 : Inport  Port=4
  Iin1 : Inport  Port=5
  In6 : Inport  Port=6
  area3 : Subsystem  mask{Subsystem=sub(3)}
      mask prompts: Subsystem "Struct"
      mask Display: disp(get_param(gcb,'Subsystem'));
  con13 : Subsystem  mask{con_subsystem=con_sub(2)}
      mask prompts: con_subsystem "Struct"
      mask Display: disp(get_param(gcb,'con_subsystem'));
  Pm_gfl3 : Outport
  Vm_gfl3 : Outport  Port=2
  Pm_gfm3 : Outport  Port=3
  Vm_gfm3 : Outport  Port=4
  Vout1 : Outport  Port=5
  Out6 : Outport  Port=6
  wires:
  con13/2(Out2) -> [Iin13_3]
  area3/5(Vout) -> [Vout3_13]
  [Vout3_13] -> con13/2(In2)
  Vr_gfm3/1 -> area3/4(Vr_gfm)
  [Iin13_3] -> area3/5(Iin)
  Vr_gfl3/1 -> area3/2(Vr_gfl)
  Pr_gfl3/1 -> area3/1(Pr_gfl)
  area3/6(Vout1) -> Vout1/1
  Pr_gfm3/1 -> area3/3(Pr_gfm)
  area3/1(Pm_gfl) -> Pm_gfl3/1
  area3/2(Vm_gfl) -> Vm_gfl3/1
  area3/4(Vm_gfm) -> Vm_gfm3/1
  area3/3(Pm_gfm) -> Pm_gfm3/1
  con13/1(Out1) -> Out6/1
  Iin1/1 -> area3/6(Iin1)
  In6/1 -> con13/1(In1)

== system subsystem_118_bus_self_clearing_blocking/Linear 118 Bus ROM/Subsystem3 ==
  Pr_gfl3 : Inport
  Vr_gfl3 : Inport  Port=2
  Pr_gfm3 : Inport  Port=3
  Vr_gfm3 : Inport  Port=4
  Iin1 : Inport  Port=5
  In6 : Inport  Port=6
  area3 : Subsystem  mask{Subsystem=sub(3)}
      mask prompts: Subsystem "Struct"
      mask Display: disp(get_param(gcb,'Subsystem'));
  con13 : Subsystem  mask{con_subsystem=con_sub(2)}
      mask prompts: con_subsystem "Struct"
      mask Display: disp(get_param(gcb,'con_subsystem'));
  Pm_gfl3 : Outport
  Vm_gfl3 : Outport  Port=2
  Pm_gfm3 : Outport  Port=3
  Vm_gfm3 : Outport  Port=4
  Vout1 : Outport  Port=5
  Out6 : Outport  Port=6
  wires:
  con13/2(Out2) -> [Iin13_3]
  area3/5(Vout) -> [Vout3_13]
  [Vout3_13] -> con13/2(In2)
  Vr_gfm3/1 -> area3/4(Vr_gfm)
  [Iin13_3] -> area3/5(Iin)
  Vr_gfl3/1 -> area3/2(Vr_gfl)
  Pr_gfl3/1 -> area3/1(Pr_gfl)
  area3/6(Vout1) -> Vout1/1
  Pr_gfm3/1 -> area3/3(Pr_gfm)
  area3/1(Pm_gfl) -> Pm_gfl3/1
  area3/2(Vm_gfl) -> Vm_gfl3/1
  area3/4(Vm_gfm) -> Vm_gfm3/1
  area3/3(Pm_gfm) -> Pm_gfm3/1
  con13/1(Out1) -> Out6/1
  Iin1/1 -> area3/6(Iin1)
  In6/1 -> con13/1(In1)

== system subsystem_118_bus_self_clearing_blocking/Subsystem1/area1 ==
  Pr_gfl : Inport  PortDimensions=max([Subsystem.n_gfl,1])
  Vr_gfl : Inport  Port=2  PortDimensions=max([Subsystem.n_gfl,1])
  Pr_gfm : Inport  Port=3  PortDimensions=max([Subsystem.n_gfm,1])
  Vr_gfm : Inport  Port=4  PortDimensions=max([Subsystem.n_gfm,1])
  Iin : Inport  Port=5
  Iin1 : Inport  Port=6
  Add : Sum  Inputs=+++
  Constant : Constant  Value=Subsystem.T
  Constant1 : Constant  Value=Subsystem.T
  Constant2 : Constant  Value=Subsystem.I_in{1}
  Constant3 : Constant  Value=Subsystem.I_in{2}
  Selector1 : Selector  InputPortWidth=size(Subsystem.sys_data,1)  IndexOptions=Index vector (dialog)  Indices=Subsystem.vout{1}'  OutputSizes=1
  Selector2 : Selector  InputPortWidth=size(Subsystem.sys_data,1)  IndexOptions=Index vector (dialog)  Indices=Subsystem.vout{2}'  OutputSizes=1
  T'x(v_bus_DQ) : Product  Multiplication=Matrix(*)
  T'x(v_bus_DQ)1 : Product  Multiplication=Matrix(*)
  T'x(v_bus_DQ)2 : Product  Multiplication=Matrix(*)
  Transpose : Math  Operator=transpose
  Tx(i_line_DQ) : Product  Multiplication=Matrix(*)
  branch RL dynamics : Subsystem
      mask Display: image('$imagefile'); % Use "Edit Image" on toolstrip to change.
  bus reordering : Subsystem
  ibr : Subsystem
      mask Display: image('$imagefile'); % Use "Edit Image" on toolstrip to change.
  non_ibr : Subsystem
      mask Display: image('$imagefile'); % Use "Edit Image" on toolstrip to change.
  Pm_gfl : Outport
  Vm_gfl : Outport  Port=2
  Pm_gfm : Outport  Port=3
  Vm_gfm : Outport  Port=4
  Vout : Outport  Port=5
  Vout1 : Outport  Port=6
  wires:
  Constant/1 -> Transpose/1
  Add/1 -> non_ibr/1(i_bus_DQ), ibr/1(I_bus_DQ)
  bus reordering/1(v_bus_DQ) -> T'x(v_bus_DQ)/2, Selector2/1, Selector1/1
  branch RL dynamics/1(i_line_DQ) -> Tx(i_line_DQ)/2
  T'x(v_bus_DQ)/1 -> branch RL dynamics/1(v_diff_DQ)
  Constant1/1 -> Tx(i_line_DQ)/1
  ibr/3(Vm) -> Vm_gfl/1
  Tx(i_line_DQ)/1 -> [i_bus_DQ]
  ibr/1(v_ibr_DQ) -> bus reordering/2(In2)
  Transpose/1 -> T'x(v_bus_DQ)/1
  non_ibr/1(v_nonibr_DQ) -> bus reordering/1(In1)
  ibr/2(Pm) -> Pm_gfl/1
  ibr/5(Vm1) -> Vm_gfm/1
  ibr/4(Pm1) -> Pm_gfm/1
  Vr_gfm/1 -> ibr/5(Inport3)
  Pr_gfm/1 -> ibr/4(Inport2)
  Vr_gfl/1 -> ibr/3(Inport1)
  Pr_gfl/1 -> ibr/2(Inport)
  Iin/1 -> T'x(v_bus_DQ)1/2
  T'x(v_bus_DQ)1/1 -> Add/1
  [i_bus_DQ] -> Add/2
  Selector1/1 -> Vout/1
  Constant2/1 -> T'x(v_bus_DQ)1/1
  Constant3/1 -> T'x(v_bus_DQ)2/1
  Iin1/1 -> T'x(v_bus_DQ)2/2
  T'x(v_bus_DQ)2/1 -> Add/3
  Selector2/1 -> Vout1/1

== system subsystem_118_bus_self_clearing_blocking/Subsystem1/con12 ==
  In1 : Inport
  In2 : Inport  Port=2
  Constant : Constant  Value=con_subsystem.T
  Constant1 : Constant  Value=con_subsystem.T
  Mux : Mux  Inputs=2
  Selector : Selector  NumberOfDimensions=2  InputPortWidth=3  IndexOptions=Index vector (dialog),Select all  Indices=con_subsystem.reorder_v',1  OutputSizes=1,1
  Selector1 : Selector  InputPortWidth=con_subsystem.nbus  IndexOptions=Index vector (dialog)  Indices=con_subsystem.I_select{1}'  OutputSizes=1
  Selector2 : Selector  InputPortWidth=con_subsystem.nbus  IndexOptions=Index vector (dialog)  Indices=con_subsystem.I_select{2}'  OutputSizes=1
  T'x(v_bus_DQ) : Product  Multiplication=Matrix(*)
  Transpose : Math  Operator=transpose
  Tx(i_line_DQ) : Product  Multiplication=Matrix(*)
  branch RL dynamics : Subsystem
      mask Display: image('$imagefile'); % Use "Edit Image" on toolstrip to change.
  Out1 : Outport
  Out2 : Outport  Port=2
  wires:
  Mux/1 -> Selector/1
  Selector/1 -> T'x(v_bus_DQ)/2
  Tx(i_line_DQ)/1 -> Selector2/1, Selector1/1
  Constant/1 -> Transpose/1
  Transpose/1 -> T'x(v_bus_DQ)/1
  Constant1/1 -> Tx(i_line_DQ)/1
  branch RL dynamics/1(i_line_DQ) -> Tx(i_line_DQ)/2
  T'x(v_bus_DQ)/1 -> branch RL dynamics/1(v_diff_DQ)
  Selector1/1 -> Out1/1
  In1/1 -> Mux/1
  Selector2/1 -> Out2/1
  In2/1 -> Mux/2

== system subsystem_118_bus_self_clearing_blocking/Subsystem2/area2 ==
  Pr_gfl : Inport  PortDimensions=max([Subsystem.n_gfl,1])
  Vr_gfl : Inport  Port=2  PortDimensions=max([Subsystem.n_gfl,1])
  Pr_gfm : Inport  Port=3  PortDimensions=max([Subsystem.n_gfm,1])
  Vr_gfm : Inport  Port=4  PortDimensions=max([Subsystem.n_gfm,1])
  Iin : Inport  Port=5
  Iin1 : Inport  Port=6
  Add : Sum  Inputs=+++
  Constant : Constant  Value=Subsystem.T
  Constant1 : Constant  Value=Subsystem.T
  Constant2 : Constant  Value=Subsystem.I_in{1}
  Constant3 : Constant  Value=Subsystem.I_in{3}
  Selector1 : Selector  InputPortWidth=size(Subsystem.sys_data,1)  IndexOptions=Index vector (dialog)  Indices=Subsystem.vout{1}'  OutputSizes=1
  Selector2 : Selector  InputPortWidth=size(Subsystem.sys_data,1)  IndexOptions=Index vector (dialog)  Indices=Subsystem.vout{3}'  OutputSizes=1
  T'x(v_bus_DQ) : Product  Multiplication=Matrix(*)
  T'x(v_bus_DQ)1 : Product  Multiplication=Matrix(*)
  T'x(v_bus_DQ)2 : Product  Multiplication=Matrix(*)
  Transpose : Math  Operator=transpose
  Tx(i_line_DQ) : Product  Multiplication=Matrix(*)
  branch RL dynamics : Subsystem
      mask Display: image('$imagefile'); % Use "Edit Image" on toolstrip to change.
  bus reordering : Subsystem
  ibr : Subsystem
      mask Display: image('$imagefile'); % Use "Edit Image" on toolstrip to change.
  non_ibr : Subsystem
      mask Display: image('$imagefile'); % Use "Edit Image" on toolstrip to change.
  Pm_gfl : Outport
  Vm_gfl : Outport  Port=2
  Pm_gfm : Outport  Port=3
  Vm_gfm : Outport  Port=4
  Vout : Outport  Port=5
  Vout1 : Outport  Port=6
  wires:
  Selector2/1 -> Vout1/1
  T'x(v_bus_DQ)2/1 -> Add/3
  Iin1/1 -> T'x(v_bus_DQ)2/2
  Constant3/1 -> T'x(v_bus_DQ)2/1
  Constant2/1 -> T'x(v_bus_DQ)1/1
  Selector1/1 -> Vout/1
  [i_bus_DQ] -> Add/2
  T'x(v_bus_DQ)1/1 -> Add/1
  Iin/1 -> T'x(v_bus_DQ)1/2
  Pr_gfl/1 -> ibr/2(Inport)
  Vr_gfl/1 -> ibr/3(Inport1)
  Pr_gfm/1 -> ibr/4(Inport2)
  Vr_gfm/1 -> ibr/5(Inport3)
  ibr/4(Pm1) -> Pm_gfm/1
  ibr/5(Vm1) -> Vm_gfm/1
  ibr/2(Pm) -> Pm_gfl/1
  non_ibr/1(v_nonibr_DQ) -> bus reordering/1(In1)
  Transpose/1 -> T'x(v_bus_DQ)/1
  ibr/1(v_ibr_DQ) -> bus reordering/2(In2)
  Tx(i_line_DQ)/1 -> [i_bus_DQ]
  ibr/3(Vm) -> Vm_gfl/1
  Constant1/1 -> Tx(i_line_DQ)/1
  T'x(v_bus_DQ)/1 -> branch RL dynamics/1(v_diff_DQ)
  branch RL dynamics/1(i_line_DQ) -> Tx(i_line_DQ)/2
  bus reordering/1(v_bus_DQ) -> Selector1/1, Selector2/1, T'x(v_bus_DQ)/2
  Add/1 -> ibr/1(I_bus_DQ), non_ibr/1(i_bus_DQ)
  Constant/1 -> Transpose/1

== system subsystem_118_bus_self_clearing_blocking/Subsystem2/con23 ==
  In1 : Inport
  In2 : Inport  Port=2
  Constant : Constant  Value=con_subsystem.T
  Constant1 : Constant  Value=con_subsystem.T
  Mux : Mux  Inputs=2
  Selector : Selector  NumberOfDimensions=2  InputPortWidth=3  IndexOptions=Index vector (dialog),Select all  Indices=con_subsystem.reorder_v',1  OutputSizes=1,1
  Selector1 : Selector  InputPortWidth=con_subsystem.nbus  IndexOptions=Index vector (dialog)  Indices=con_subsystem.I_select{2}'  OutputSizes=1
  Selector2 : Selector  InputPortWidth=con_subsystem.nbus  IndexOptions=Index vector (dialog)  Indices=con_subsystem.I_select{3}'  OutputSizes=1
  T'x(v_bus_DQ) : Product  Multiplication=Matrix(*)
  Transpose : Math  Operator=transpose
  Tx(i_line_DQ) : Product  Multiplication=Matrix(*)
  branch RL dynamics : Subsystem
      mask Display: image('$imagefile'); % Use "Edit Image" on toolstrip to change.
  Out1 : Outport
  Out2 : Outport  Port=2
  wires:
  Mux/1 -> Selector/1
  Selector/1 -> T'x(v_bus_DQ)/2
  Tx(i_line_DQ)/1 -> Selector2/1, Selector1/1
  Constant/1 -> Transpose/1
  Transpose/1 -> T'x(v_bus_DQ)/1
  Constant1/1 -> Tx(i_line_DQ)/1
  branch RL dynamics/1(i_line_DQ) -> Tx(i_line_DQ)/2
  T'x(v_bus_DQ)/1 -> branch RL dynamics/1(v_diff_DQ)
  Selector1/1 -> Out1/1
  In1/1 -> Mux/1
  Selector2/1 -> Out2/1
  In2/1 -> Mux/2

== system subsystem_118_bus_self_clearing_blocking/Subsystem3/area3 ==
  Pr_gfl : Inport  PortDimensions=max([Subsystem.n_gfl,1])
  Vr_gfl : Inport  Port=2  PortDimensions=max([Subsystem.n_gfl,1])
  Pr_gfm : Inport  Port=3  PortDimensions=max([Subsystem.n_gfm,1])
  Vr_gfm : Inport  Port=4  PortDimensions=max([Subsystem.n_gfm,1])
  Iin : Inport  Port=5
  Iin1 : Inport  Port=6
  Add : Sum  Inputs=+++
  Constant : Constant  Value=Subsystem.T
  Constant1 : Constant  Value=Subsystem.T
  Constant2 : Constant  Value=Subsystem.I_in{2}
  Constant3 : Constant  Value=Subsystem.I_in{3}
  Selector1 : Selector  InputPortWidth=size(Subsystem.sys_data,1)  IndexOptions=Index vector (dialog)  Indices=Subsystem.vout{2}'  OutputSizes=1
  Selector2 : Selector  InputPortWidth=size(Subsystem.sys_data,1)  IndexOptions=Index vector (dialog)  Indices=Subsystem.vout{3}'  OutputSizes=1
  T'x(v_bus_DQ) : Product  Multiplication=Matrix(*)
  T'x(v_bus_DQ)1 : Product  Multiplication=Matrix(*)
  T'x(v_bus_DQ)2 : Product  Multiplication=Matrix(*)
  Transpose : Math  Operator=transpose
  Tx(i_line_DQ) : Product  Multiplication=Matrix(*)
  branch RL dynamics : Subsystem
      mask Display: image('$imagefile'); % Use "Edit Image" on toolstrip to change.
  bus reordering : Subsystem
  ibr : Subsystem
      mask Display: image('$imagefile'); % Use "Edit Image" on toolstrip to change.
  non_ibr : Subsystem
      mask Display: image('$imagefile'); % Use "Edit Image" on toolstrip to change.
  Pm_gfl : Outport
  Vm_gfl : Outport  Port=2
  Pm_gfm : Outport  Port=3
  Vm_gfm : Outport  Port=4
  Vout : Outport  Port=5
  Vout1 : Outport  Port=6
  wires:
  Constant/1 -> Transpose/1
  Add/1 -> ibr/1(I_bus_DQ), non_ibr/1(i_bus_DQ)
  bus reordering/1(v_bus_DQ) -> T'x(v_bus_DQ)/2, Selector2/1, Selector1/1
  branch RL dynamics/1(i_line_DQ) -> Tx(i_line_DQ)/2
  T'x(v_bus_DQ)/1 -> branch RL dynamics/1(v_diff_DQ)
  Constant1/1 -> Tx(i_line_DQ)/1
  ibr/3(Vm) -> Vm_gfl/1
  Tx(i_line_DQ)/1 -> [i_bus_DQ]
  ibr/1(v_ibr_DQ) -> bus reordering/2(In2)
  Transpose/1 -> T'x(v_bus_DQ)/1
  non_ibr/1(v_nonibr_DQ) -> bus reordering/1(In1)
  ibr/2(Pm) -> Pm_gfl/1
  ibr/5(Vm1) -> Vm_gfm/1
  ibr/4(Pm1) -> Pm_gfm/1
  Vr_gfm/1 -> ibr/5(Inport3)
  Pr_gfm/1 -> ibr/4(Inport2)
  Vr_gfl/1 -> ibr/3(Inport1)
  Pr_gfl/1 -> ibr/2(Inport)
  Iin/1 -> T'x(v_bus_DQ)1/2
  T'x(v_bus_DQ)1/1 -> Add/1
  [i_bus_DQ] -> Add/2
  Selector1/1 -> Vout/1
  Constant2/1 -> T'x(v_bus_DQ)1/1
  Constant3/1 -> T'x(v_bus_DQ)2/1
  Iin1/1 -> T'x(v_bus_DQ)2/2
  T'x(v_bus_DQ)2/1 -> Add/3
  Selector2/1 -> Vout1/1

== system subsystem_118_bus_self_clearing_blocking/Subsystem3/con13 ==
  In1 : Inport
  In2 : Inport  Port=2
  Constant : Constant  Value=con_subsystem.T
  Constant1 : Constant  Value=con_subsystem.T
  Mux : Mux  Inputs=2
  Selector : Selector  NumberOfDimensions=2  InputPortWidth=3  IndexOptions=Index vector (dialog),Select all  Indices=con_subsystem.reorder_v',1  OutputSizes=1,1
  Selector1 : Selector  InputPortWidth=con_subsystem.nbus  IndexOptions=Index vector (dialog)  Indices=con_subsystem.I_select{1}'  OutputSizes=1
  Selector2 : Selector  InputPortWidth=con_subsystem.nbus  IndexOptions=Index vector (dialog)  Indices=con_subsystem.I_select{3}'  OutputSizes=1
  T'x(v_bus_DQ) : Product  Multiplication=Matrix(*)
  Transpose : Math  Operator=transpose
  Tx(i_line_DQ) : Product  Multiplication=Matrix(*)
  branch RL dynamics : Subsystem
      mask Display: image('$imagefile'); % Use "Edit Image" on toolstrip to change.
  Out1 : Outport
  Out2 : Outport  Port=2
  wires:
  In2/1 -> Mux/2
  Selector2/1 -> Out2/1
  In1/1 -> Mux/1
  Selector1/1 -> Out1/1
  T'x(v_bus_DQ)/1 -> branch RL dynamics/1(v_diff_DQ)
  branch RL dynamics/1(i_line_DQ) -> Tx(i_line_DQ)/2
  Constant1/1 -> Tx(i_line_DQ)/1
  Transpose/1 -> T'x(v_bus_DQ)/1
  Constant/1 -> Transpose/1
  Tx(i_line_DQ)/1 -> Selector1/1, Selector2/1
  Selector/1 -> T'x(v_bus_DQ)/2
  Mux/1 -> Selector/1

== system subsystem_118_bus_self_clearing_blocking/Linear 118 Bus FOM/Subsystem3/area3 ==
  Pr_gfl : Inport  PortDimensions=max([Subsystem.n_gfl,1])
  Vr_gfl : Inport  Port=2  PortDimensions=max([Subsystem.n_gfl,1])
  Pr_gfm : Inport  Port=3  PortDimensions=max([Subsystem.n_gfm,1])
  Vr_gfm : Inport  Port=4  PortDimensions=max([Subsystem.n_gfm,1])
  Iin : Inport  Port=5
  Iin1 : Inport  Port=6
  Add : Sum  Inputs=+++
  Constant : Constant  Value=Subsystem.T
  Constant1 : Constant  Value=Subsystem.T
  Constant2 : Constant  Value=Subsystem.I_in{2}
  Constant3 : Constant  Value=Subsystem.I_in{3}
  Selector1 : Selector  InputPortWidth=size(Subsystem.sys_data,1)  IndexOptions=Index vector (dialog)  Indices=Subsystem.vout{2}'  OutputSizes=1
  Selector2 : Selector  InputPortWidth=size(Subsystem.sys_data,1)  IndexOptions=Index vector (dialog)  Indices=Subsystem.vout{3}'  OutputSizes=1
  T'x(v_bus_DQ) : Product  Multiplication=Matrix(*)
  T'x(v_bus_DQ)1 : Product  Multiplication=Matrix(*)
  T'x(v_bus_DQ)2 : Product  Multiplication=Matrix(*)
  Transpose : Math  Operator=transpose
  Tx(i_line_DQ) : Product  Multiplication=Matrix(*)
  branch RL dynamics : Subsystem
      mask Display: image('$imagefile'); % Use "Edit Image" on toolstrip to change.
  bus reordering : Subsystem
  ibr : Subsystem
      mask Display: image('$imagefile'); % Use "Edit Image" on toolstrip to change.
  non_ibr : Subsystem
      mask Display: image('$imagefile'); % Use "Edit Image" on toolstrip to change.
  Pm_gfl : Outport
  Vm_gfl : Outport  Port=2
  Pm_gfm : Outport  Port=3
  Vm_gfm : Outport  Port=4
  Vout : Outport  Port=5
  Vout1 : Outport  Port=6
  wires:
  Constant/1 -> Transpose/1
  Add/1 -> ibr/1(I_bus_DQ), non_ibr/1(i_bus_DQ)
  bus reordering/1(v_bus_DQ) -> T'x(v_bus_DQ)/2, Selector2/1, Selector1/1
  branch RL dynamics/1(i_line_DQ) -> Tx(i_line_DQ)/2
  T'x(v_bus_DQ)/1 -> branch RL dynamics/1(v_diff_DQ)
  Constant1/1 -> Tx(i_line_DQ)/1
  ibr/3(Vm) -> Vm_gfl/1
  Tx(i_line_DQ)/1 -> [i_bus_DQ]
  ibr/1(v_ibr_DQ) -> bus reordering/2(In2)
  Transpose/1 -> T'x(v_bus_DQ)/1
  non_ibr/1(v_nonibr_DQ) -> bus reordering/1(In1)
  ibr/2(Pm) -> Pm_gfl/1
  ibr/5(Vm1) -> Vm_gfm/1
  ibr/4(Pm1) -> Pm_gfm/1
  Vr_gfm/1 -> ibr/5(Inport3)
  Pr_gfm/1 -> ibr/4(Inport2)
  Vr_gfl/1 -> ibr/3(Inport1)
  Pr_gfl/1 -> ibr/2(Inport)
  Iin/1 -> T'x(v_bus_DQ)1/2
  T'x(v_bus_DQ)1/1 -> Add/1
  [i_bus_DQ] -> Add/2
  Selector1/1 -> Vout/1
  Constant2/1 -> T'x(v_bus_DQ)1/1
  Constant3/1 -> T'x(v_bus_DQ)2/1
  Iin1/1 -> T'x(v_bus_DQ)2/2
  T'x(v_bus_DQ)2/1 -> Add/3
  Selector2/1 -> Vout1/1
